simulink model "Greska"  (R2016b)
settings: Solver=VariableStepAuto  StartTime=0.0  StopTime=800  RelTol=1e-3
libraries: simulink x2
settings Model: Creator=Luka  LastModifiedBy=Luka

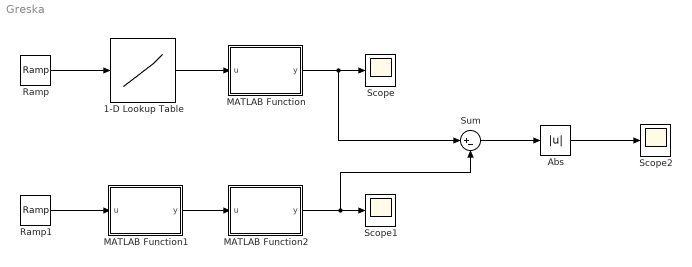
== system Greska ==
  1-D Lookup Table : Lookup_n-D  NumberOfTableDimensions=1  BreakpointsForDimension1=[0 100 200 300 400 500 600 700 800]  Table=[0 19.673 31.606 38.843 43.233 45.896 47.511 48.490 49.084]  InternalRulePriority=Speed  RndMeth=Simplest  InputSameDT=on
  Abs : Abs
  MATLAB Function : MATLAB Function  TreatAsAtomicUnit=on
  MATLAB Function1 : MATLAB Function  TreatAsAtomicUnit=on
  MATLAB Function2 : MATLAB Function  TreatAsAtomicUnit=on
  Ramp : simulink/Sources/Ramp  slope=1  start=0  X0=0
  Ramp1 : simulink/Sources/Ramp  slope=1  start=0  X0=0
  Scope : Scope
  Scope1 : Scope
  Scope2 : Scope
  Sum : Sum  Inputs=|+-
  wires:
  1-D Lookup Table/1 -> MATLAB Function/1(u)
  MATLAB Function/1(y) -> Sum/1, Scope/1
  MATLAB Function2/1(y) -> Sum/2, Scope1/1
  Abs/1 -> Scope2/1
  MATLAB Function1/1(y) -> MATLAB Function2/1(u)
  Ramp/1 -> 1-D Lookup Table/1
  Ramp1/1 -> MATLAB Function1/1(u)
  Sum/1 -> Abs/1

== matlab function Greska/MATLAB Function1 ==
  data: u input; y output
function y = fcn(u)

y = 50*(1-exp(-0.005*u));

== matlab function Greska/MATLAB Function ==
  data: u input; y output
function y = fcn(u)

y = -200*log(1 - u/50);

== matlab function Greska/MATLAB Function2 ==
  data: u input; y output
function y = fcn(u)

y = -200*log(1 - u/50);
